simulink model "myproject_task"  (Simulink 3.00)
libraries: mathlib x20, logiclib x14, inoutlib x9, execlib x4, genlib x2

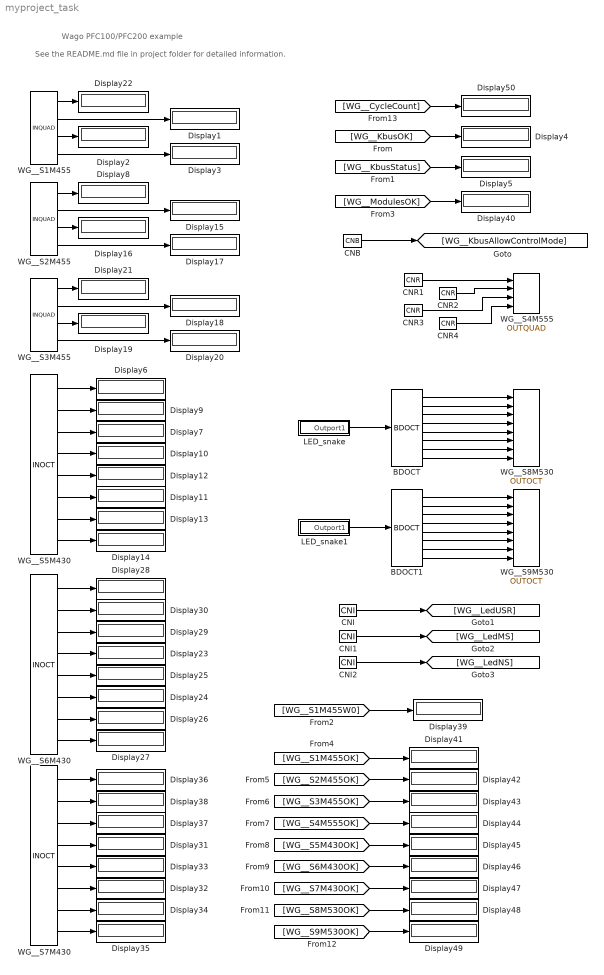
== system myproject_task ==
  note: See the README.md file in project folder for detailed information.
  note: Wago PFC100/PFC200 example
  BDOCT : logiclib/BDOCT  shift=0
  BDOCT1 : logiclib/BDOCT  shift=0
  CNB : mathlib/CNB  YCN=off
  CNI : mathlib/CNI  icn=0
  CNI1 : mathlib/CNI  icn=0
  CNI2 : mathlib/CNI  icn=0
  CNR{1..4} (4 alike) : mathlib/CNR  ycn=0
  Display{1..50} (50 alike) : Display
      Display1 settings: Format=short
      Display10 settings: Format=Best fit
      Display11 settings: Format=Best fit
      Display12 settings: Format=Best fit
      Display13 settings: Format=Best fit
      Display14 settings: Format=Best fit
      Display15 settings: Format=short
      Display16 settings: Format=short
      Display17 settings: Format=short
      Display18 settings: Format=short
      Display19 settings: Format=short
      Display2 settings: Format=short
      Display20 settings: Format=short
      Display21 settings: Format=short
      Display22 settings: Format=short
      Display23 settings: Format=Best fit
      Display24 settings: Format=Best fit
      Display25 settings: Format=Best fit
      Display26 settings: Format=Best fit
      Display27 settings: Format=Best fit
      Display28 settings: Format=Best fit
      Display29 settings: Format=Best fit
      Display3 settings: Format=short
      Display30 settings: Format=Best fit
      Display31 settings: Format=Best fit
      Display32 settings: Format=Best fit
      Display33 settings: Format=Best fit
      Display34 settings: Format=Best fit
      Display35 settings: Format=Best fit
      Display36 settings: Format=Best fit
      Display37 settings: Format=Best fit
      Display38 settings: Format=Best fit
      Display39 settings: Format=bin
      Display4 settings: Format=Best fit
      Display40 settings: Format=Best fit
      Display41 settings: Format=Best fit
      Display42 settings: Format=Best fit
      Display43 settings: Format=Best fit
      Display44 settings: Format=Best fit
      Display45 settings: Format=Best fit
      Display46 settings: Format=Best fit
      Display47 settings: Format=Best fit
      Display48 settings: Format=Best fit
      Display49 settings: Format=Best fit
      Display5 settings: Format=Best fit
      Display50 settings: Format=Best fit
      Display6 settings: Format=Best fit
      Display7 settings: Format=Best fit
      Display8 settings: Format=short
      Display9 settings: Format=Best fit
  LED_snake : Subsystem
      mask Type: REX sequence
  LED_snake1 : Subsystem
      mask Type: REX sequence
  WG__S1M455 : inoutlib/INQUAD
  WG__S2M455 : inoutlib/INQUAD
  WG__S3M455 : inoutlib/INQUAD
  WG__S4M555 : inoutlib/OUTQUAD
  WG__S5M430 : inoutlib/INOCT
  WG__S6M430 : inoutlib/INOCT
  WG__S7M430 : inoutlib/INOCT
  WG__S8M530 : inoutlib/OUTOCT
  WG__S9M530 : inoutlib/OUTOCT
  wires:
  BDOCT/1 -> WG__S8M530/1
  BDOCT/2 -> WG__S8M530/2
  BDOCT/3 -> WG__S8M530/3
  BDOCT/4 -> WG__S8M530/4
  BDOCT/5 -> WG__S8M530/5
  BDOCT/6 -> WG__S8M530/6
  BDOCT/7 -> WG__S8M530/7
  BDOCT/8 -> WG__S8M530/8
  BDOCT1/1 -> WG__S9M530/1
  BDOCT1/2 -> WG__S9M530/2
  BDOCT1/3 -> WG__S9M530/3
  BDOCT1/4 -> WG__S9M530/4
  BDOCT1/5 -> WG__S9M530/5
  BDOCT1/6 -> WG__S9M530/6
  BDOCT1/7 -> WG__S9M530/7
  BDOCT1/8 -> WG__S9M530/8
  CNB/1 -> [WG__KbusAllowControlMode]
  CNI/1 -> [WG__LedUSR]
  CNI1/1 -> [WG__LedMS]
  CNI2/1 -> [WG__LedNS]
  CNR1/1 -> WG__S4M555/1
  CNR2/1 -> WG__S4M555/2
  CNR3/1 -> WG__S4M555/3
  CNR4/1 -> WG__S4M555/4
  [WG__KbusOK] -> Display4/1
  [WG__KbusStatus] -> Display5/1
  [WG__S7M430OK] -> Display47/1
  [WG__S8M530OK] -> Display48/1
  [WG__S9M530OK] -> Display49/1
  [WG__CycleCount] -> Display50/1
  [WG__S1M455W0] -> Display39/1
  [WG__ModulesOK] -> Display40/1
  [WG__S1M455OK] -> Display41/1
  [WG__S2M455OK] -> Display42/1
  [WG__S3M455OK] -> Display43/1
  [WG__S4M555OK] -> Display44/1
  [WG__S5M430OK] -> Display45/1
  [WG__S6M430OK] -> Display46/1
  LED_snake/1(Outport1) -> BDOCT/1
  LED_snake1/1(Outport1) -> BDOCT1/1
  WG__S1M455/1 -> Display22/1
  WG__S1M455/2 -> Display1/1
  WG__S1M455/3 -> Display2/1
  WG__S1M455/4 -> Display3/1
  WG__S2M455/1 -> Display8/1
  WG__S2M455/2 -> Display15/1
  WG__S2M455/3 -> Display16/1
  WG__S2M455/4 -> Display17/1
  WG__S3M455/1 -> Display21/1
  WG__S3M455/2 -> Display18/1
  WG__S3M455/3 -> Display19/1
  WG__S3M455/4 -> Display20/1
  WG__S5M430/1 -> Display6/1
  WG__S5M430/2 -> Display9/1
  WG__S5M430/3 -> Display7/1
  WG__S5M430/4 -> Display10/1
  WG__S5M430/5 -> Display12/1
  WG__S5M430/6 -> Display11/1
  WG__S5M430/7 -> Display13/1
  WG__S5M430/8 -> Display14/1
  WG__S6M430/1 -> Display28/1
  WG__S6M430/2 -> Display30/1
  WG__S6M430/3 -> Display29/1
  WG__S6M430/4 -> Display23/1
  WG__S6M430/5 -> Display25/1
  WG__S6M430/6 -> Display24/1
  WG__S6M430/7 -> Display26/1
  WG__S6M430/8 -> Display27/1
  WG__S7M430/1 -> Display36/1
  WG__S7M430/2 -> Display38/1
  WG__S7M430/3 -> Display37/1
  WG__S7M430/4 -> Display31/1
  WG__S7M430/5 -> Display33/1
  WG__S7M430/6 -> Display32/1
  WG__S7M430/7 -> Display34/1
  WG__S7M430/8 -> Display35/1

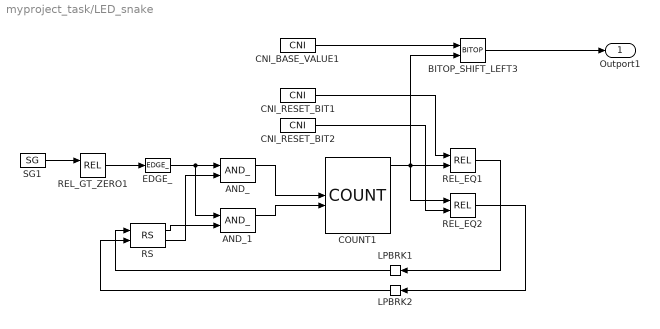
== system myproject_task/LED_snake ==
  AND_ : logiclib/AND_
  AND_1 : logiclib/AND_
  BITOP_SHIFT_LEFT3 : logiclib/BITOP  iop=5: Shift Left
  CNI_BASE_VALUE1 : mathlib/CNI  icn=1
  CNI_RESET_BIT1 : mathlib/CNI  icn=7
  CNI_RESET_BIT2 : mathlib/CNI  icn=0
  COUNT1 : logiclib/COUNT
  EDGE_ : logiclib/EDGE_  iedge=1: Rising edge
  LPBRK1 : execlib/LPBRK  Orientation=left
  LPBRK2 : execlib/LPBRK  Orientation=left
  REL_EQ1 : mathlib/REL  irel=1: equality (==)
  REL_EQ2 : mathlib/REL  irel=1: equality (==)
  REL_GT_ZERO1 : mathlib/REL  irel=4: greater than (>)
  RS : logiclib/RS
  SG1 : genlib/SG  isig=2: SQUARE  amp=1.0000000E+000  freq=10  phase=0.0000000E+000  ifrunit=1: Hz  iphunit=1: degrees  offset=0
  Outport1 : Outport  Port=1  offset=0
  wires:
  AND_/1 -> COUNT1/4
  AND_1/1 -> COUNT1/5
  BITOP_SHIFT_LEFT3/1 -> Outport1/1
  CNI_BASE_VALUE1/1 -> BITOP_SHIFT_LEFT3/1
  CNI_RESET_BIT1/1 -> REL_EQ1/1
  CNI_RESET_BIT2/1 -> REL_EQ2/2
  COUNT1/1 -> BITOP_SHIFT_LEFT3/2, REL_EQ1/2, REL_EQ2/1
  EDGE_/1 -> AND_/1, AND_1/1
  LPBRK1/1 -> RS/1
  LPBRK2/1 -> RS/2
  REL_EQ1/1 -> LPBRK1/1
  REL_EQ2/1 -> LPBRK2/1
  REL_GT_ZERO1/1 -> EDGE_/1
  RS/1 -> AND_1/2
  RS/2 -> AND_/2
  SG1/1 -> REL_GT_ZERO1/1

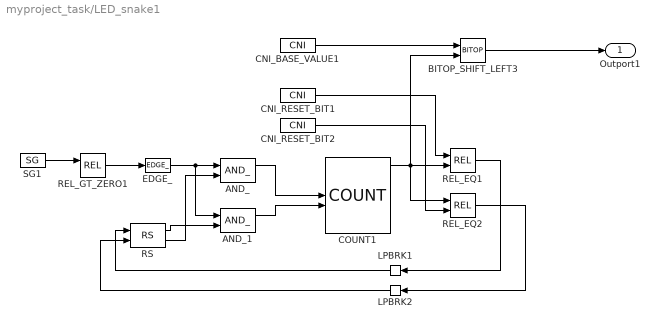
== system myproject_task/LED_snake1 ==
  AND_ : logiclib/AND_
  AND_1 : logiclib/AND_
  BITOP_SHIFT_LEFT3 : logiclib/BITOP  iop=5: Shift Left
  CNI_BASE_VALUE1 : mathlib/CNI  icn=1
  CNI_RESET_BIT1 : mathlib/CNI  icn=7
  CNI_RESET_BIT2 : mathlib/CNI  icn=0
  COUNT1 : logiclib/COUNT
  EDGE_ : logiclib/EDGE_  iedge=1: Rising edge
  LPBRK1 : execlib/LPBRK  Orientation=left
  LPBRK2 : execlib/LPBRK  Orientation=left
  REL_EQ1 : mathlib/REL  irel=1: equality (==)
  REL_EQ2 : mathlib/REL  irel=1: equality (==)
  REL_GT_ZERO1 : mathlib/REL  irel=4: greater than (>)
  RS : logiclib/RS
  SG1 : genlib/SG  isig=2: SQUARE  amp=1.0000000E+000  freq=10  phase=0.0000000E+000  ifrunit=1: Hz  iphunit=1: degrees  offset=0
  Outport1 : Outport  Port=1  offset=0
  wires:
  AND_/1 -> COUNT1/4
  AND_1/1 -> COUNT1/5
  BITOP_SHIFT_LEFT3/1 -> Outport1/1
  CNI_BASE_VALUE1/1 -> BITOP_SHIFT_LEFT3/1
  CNI_RESET_BIT1/1 -> REL_EQ1/1
  CNI_RESET_BIT2/1 -> REL_EQ2/2
  COUNT1/1 -> BITOP_SHIFT_LEFT3/2, REL_EQ1/2, REL_EQ2/1
  EDGE_/1 -> AND_/1, AND_1/1
  LPBRK1/1 -> RS/1
  LPBRK2/1 -> RS/2
  REL_EQ1/1 -> LPBRK1/1
  REL_EQ2/1 -> LPBRK2/1
  REL_GT_ZERO1/1 -> EDGE_/1
  RS/1 -> AND_1/2
  RS/2 -> AND_/2
  SG1/1 -> REL_GT_ZERO1/1
